simulink model "OL_HiLData"  (R2015b)
settings: Solver=FixedStepDiscrete  StartTime=0.0  StopTime=stop_time  FixedStep=step_size  RelTol=1e-3
values from neighbouring files (symbols this model uses):
  step_size = 0.1    [loadCalib.m]
  stop_time = 660    [run_test_cases.m]
undefined symbols (not defined in the file or in its folder): canChannel
libraries: canmsglib x62, canlib x29, realtime_pacer_lib x1
(part 4 of 4)

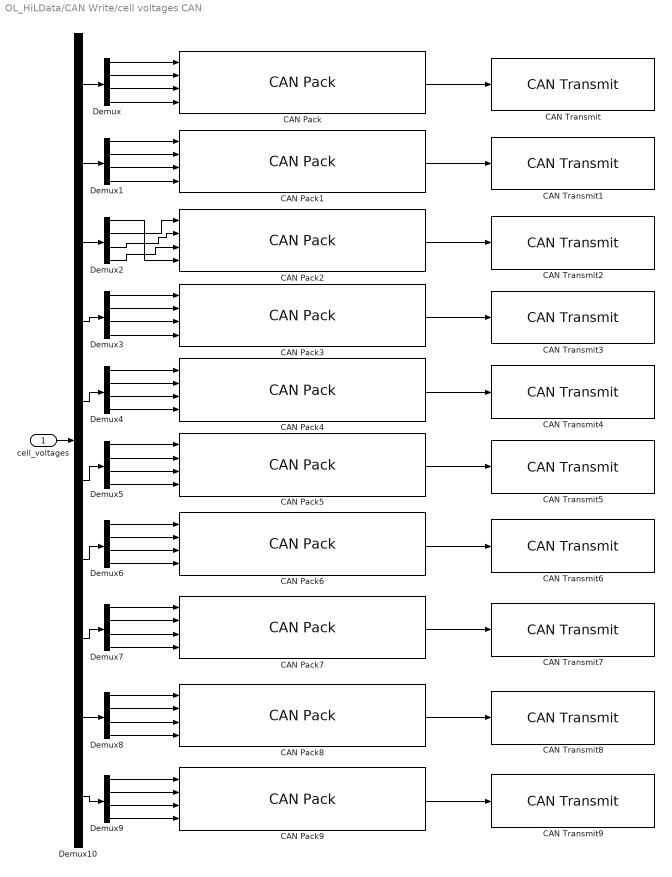
== system OL_HiLData/CAN Write/cell voltages CAN ==
  cell_voltages : Inport
  CAN Pack : canmsglib/CAN Pack  CANdbFile=D:\Projects\BMS\P006n\08_Work_in_progress\Repo_Sync_folder\OpenLoopDataSendCAN\BMSdb.dbc  MsgList=cell_voltage_1_4  MsgName=cell_voltage_1_4  MsgIDType=Standard (11-bit identifier)  MsgIdentifier=2  MsgLength=8  SignalInfo=cell1_voltage$8$16$2$2$1$0$1.000000e-04$0$0$5$#cell2_voltage$24$16$2$2$1$0$1.000000e-04$0$0$5$#cell3_voltage$40$16$2$2$1$0$1.000000e-04$0$0$5$#cell4_voltage$56$16$2$2$1$0$1.000000e-04$0$0$5$#  NSignals=4  StartBits=str2num('[int32(8);int32(24);int32(40);int32(56)]')  SignalSizes=str2num('[int32(16);int32(16);int32(16);int32(16)]')  ByteOrders=str2num('[int32(2);int32(2);int32(2);int32(2)]')  DataTypes=str2num('[int32(2);int32(2);int32(2);int32(2)]')  MultiplexTypes=str2num('[int32(1);int32(1);int32(1);int32(1)]')  MultiplexValues=str2num('[double(0);double(0);double(0);double(0)]')  Factors=str2num('[double(1.000000e-04);double(1.000000e-04);double(1.000000e-04);double(1.000000e-04)]')  Offsets=str2num('[double(0);double(0);double(0);double(0)]')  Minimums=str2num('[double(0);double(0);double(0);double(0)]')  Maximums=str2num('[double(5);double(5);double(5);double(5)]')  Remote=off
      settings: DataFormat=CANdb specified signals
  CAN Pack1 : canmsglib/CAN Pack  CANdbFile=D:\Projects\BMS\P006n\08_Work_in_progress\Repo_Sync_folder\OpenLoopDataSendCAN\BMSdb.dbc  MsgList=cell_voltage_5_8  MsgName=cell_voltage_5_8  MsgIDType=Standard (11-bit identifier)  MsgIdentifier=3  MsgLength=8  SignalInfo=cell5_votlage$8$16$2$2$1$0$1.000000e-04$0$0$5$#cell6_voltage$24$16$2$2$1$0$1.000000e-04$0$0$5$#cell7_voltage$40$16$2$2$1$0$1.000000e-04$0$0$5$#cell8_voltage$56$16$2$2$1$0$1.000000e-04$0$0$5$#  NSignals=4  StartBits=str2num('[int32(8);int32(24);int32(40);int32(56)]')  SignalSizes=str2num('[int32(16);int32(16);int32(16);int32(16)]')  ByteOrders=str2num('[int32(2);int32(2);int32(2);int32(2)]')  DataTypes=str2num('[int32(2);int32(2);int32(2);int32(2)]')  MultiplexTypes=str2num('[int32(1);int32(1);int32(1);int32(1)]')  MultiplexValues=str2num('[double(0);double(0);double(0);double(0)]')  Factors=str2num('[double(1.000000e-04);double(1.000000e-04);double(1.000000e-04);double(1.000000e-04)]')  Offsets=str2num('[double(0);double(0);double(0);double(0)]')  Minimums=str2num('[double(0);double(0);double(0);double(0)]')  Maximums=str2num('[double(5);double(5);double(5);double(5)]')  Remote=off
      settings: DataFormat=CANdb specified signals
  CAN Pack2 : canmsglib/CAN Pack  CANdbFile=D:\Projects\BMS\P006n\08_Work_in_progress\Repo_Sync_folder\OpenLoopDataSendCAN\BMSdb.dbc  MsgList=cell_voltage_9_12  MsgName=cell_voltage_9_12  MsgIDType=Standard (11-bit identifier)  MsgIdentifier=4  MsgLength=8  SignalInfo=cell10_voltage$24$16$2$2$1$0$1.000000e-04$0$0$5$#cell11_voltage$40$16$2$2$1$0$1.000000e-04$0$0$5$#cell12_voltage$56$16$2$2$1$0$1.000000e-04$0$0$5$#cell9_votlage$8$16$2$2$1$0$1.000000e-04$0$0$5$#  NSignals=4  StartBits=str2num('[int32(24);int32(40);int32(56);int32(8)]')  SignalSizes=str2num('[int32(16);int32(16);int32(16);int32(16)]')  ByteOrders=str2num('[int32(2);int32(2);int32(2);int32(2)]')  DataTypes=str2num('[int32(2);int32(2);int32(2);int32(2)]')  MultiplexTypes=str2num('[int32(1);int32(1);int32(1);int32(1)]')  MultiplexValues=str2num('[double(0);double(0);double(0);double(0)]')  Factors=str2num('[double(1.000000e-04);double(1.000000e-04);double(1.000000e-04);double(1.000000e-04)]')  Offsets=str2num('[double(0);double(0);double(0);double(0)]')  Minimums=str2num('[double(0);double(0);double(0);double(0)]')  Maximums=str2num('[double(5);double(5);double(5);double(5)]')  Remote=off
      settings: DataFormat=CANdb specified signals
  CAN Pack3 : canmsglib/CAN Pack  CANdbFile=D:\Projects\BMS\P006n\08_Work_in_progress\Repo_Sync_folder\OpenLoopDataSendCAN\BMSdb.dbc  MsgList=cell_voltage_13_16  MsgName=cell_voltage_13_16  MsgIDType=Standard (11-bit identifier)  MsgIdentifier=5  MsgLength=8  SignalInfo=cell13_votlage$8$16$2$2$1$0$1.000000e-04$0$0$5$#cell14_voltage$24$16$2$2$1$0$1.000000e-04$0$0$5$#cell15_voltage$40$16$2$2$1$0$1.000000e-04$0$0$5$#cell16_voltage$56$16$2$2$1$0$1.000000e-04$0$0$5$#  NSignals=4  StartBits=str2num('[int32(8);int32(24);int32(40);int32(56)]')  SignalSizes=str2num('[int32(16);int32(16);int32(16);int32(16)]')  ByteOrders=str2num('[int32(2);int32(2);int32(2);int32(2)]')  DataTypes=str2num('[int32(2);int32(2);int32(2);int32(2)]')  MultiplexTypes=str2num('[int32(1);int32(1);int32(1);int32(1)]')  MultiplexValues=str2num('[double(0);double(0);double(0);double(0)]')  Factors=str2num('[double(1.000000e-04);double(1.000000e-04);double(1.000000e-04);double(1.000000e-04)]')  Offsets=str2num('[double(0);double(0);double(0);double(0)]')  Minimums=str2num('[double(0);double(0);double(0);double(0)]')  Maximums=str2num('[double(5);double(5);double(5);double(5)]')  Remote=off
      settings: DataFormat=CANdb specified signals
  CAN Pack4 : canmsglib/CAN Pack  CANdbFile=D:\Projects\BMS\P006n\08_Work_in_progress\Repo_Sync_folder\OpenLoopDataSendCAN\BMSdb.dbc  MsgList=cell_voltage_17_20  MsgName=cell_voltage_17_20  MsgIDType=Standard (11-bit identifier)  MsgIdentifier=6  MsgLength=8  SignalInfo=cell17_votlage$8$16$2$2$1$0$1.000000e-04$0$0$5$#cell18_voltage$24$16$2$2$1$0$1.000000e-04$0$0$5$#cell19_voltage$40$16$2$2$1$0$1.000000e-04$0$0$5$#cell20_voltage$56$16$2$2$1$0$1.000000e-04$0$0$5$#  NSignals=4  StartBits=str2num('[int32(8);int32(24);int32(40);int32(56)]')  SignalSizes=str2num('[int32(16);int32(16);int32(16);int32(16)]')  ByteOrders=str2num('[int32(2);int32(2);int32(2);int32(2)]')  DataTypes=str2num('[int32(2);int32(2);int32(2);int32(2)]')  MultiplexTypes=str2num('[int32(1);int32(1);int32(1);int32(1)]')  MultiplexValues=str2num('[double(0);double(0);double(0);double(0)]')  Factors=str2num('[double(1.000000e-04);double(1.000000e-04);double(1.000000e-04);double(1.000000e-04)]')  Offsets=str2num('[double(0);double(0);double(0);double(0)]')  Minimums=str2num('[double(0);double(0);double(0);double(0)]')  Maximums=str2num('[double(5);double(5);double(5);double(5)]')  Remote=off
      settings: DataFormat=CANdb specified signals
  CAN Pack5 : canmsglib/CAN Pack  CANdbFile=D:\Projects\BMS\P006n\08_Work_in_progress\Repo_Sync_folder\OpenLoopDataSendCAN\BMSdb.dbc  MsgList=cell_voltage_21_24  MsgName=cell_voltage_21_24  MsgIDType=Standard (11-bit identifier)  MsgIdentifier=7  MsgLength=8  SignalInfo=cell21_votlage$8$16$2$2$1$0$1.000000e-04$0$0$5$#cell22_votlage$24$16$2$2$1$0$1.000000e-04$0$0$5$#cell23_votlage$40$16$2$2$1$0$1.000000e-04$0$0$5$#cell24_votlage$56$16$2$2$1$0$1.000000e-04$0$0$5$#  NSignals=4  StartBits=str2num('[int32(8);int32(24);int32(40);int32(56)]')  SignalSizes=str2num('[int32(16);int32(16);int32(16);int32(16)]')  ByteOrders=str2num('[int32(2);int32(2);int32(2);int32(2)]')  DataTypes=str2num('[int32(2);int32(2);int32(2);int32(2)]')  MultiplexTypes=str2num('[int32(1);int32(1);int32(1);int32(1)]')  MultiplexValues=str2num('[double(0);double(0);double(0);double(0)]')  Factors=str2num('[double(1.000000e-04);double(1.000000e-04);double(1.000000e-04);double(1.000000e-04)]')  Offsets=str2num('[double(0);double(0);double(0);double(0)]')  Minimums=str2num('[double(0);double(0);double(0);double(0)]')  Maximums=str2num('[double(5);double(5);double(5);double(5)]')  Remote=off
      settings: DataFormat=CANdb specified signals
  CAN Pack6 : canmsglib/CAN Pack  CANdbFile=D:\Projects\BMS\P006n\08_Work_in_progress\Repo_Sync_folder\OpenLoopDataSendCAN\BMSdb.dbc  MsgList=cell_voltage_25_28  MsgName=cell_voltage_25_28  MsgIDType=Standard (11-bit identifier)  MsgIdentifier=8  MsgLength=8  SignalInfo=cell25_votlage$8$16$2$2$1$0$1.000000e-04$0$0$5$#cell26_votlage$24$16$2$2$1$0$1.000000e-04$0$0$5$#cell27_votlage$40$16$2$2$1$0$1.000000e-04$0$0$5$#cell28_votlage$56$16$2$2$1$0$1.000000e-04$0$0$5$#  NSignals=4  StartBits=str2num('[int32(8);int32(24);int32(40);int32(56)]')  SignalSizes=str2num('[int32(16);int32(16);int32(16);int32(16)]')  ByteOrders=str2num('[int32(2);int32(2);int32(2);int32(2)]')  DataTypes=str2num('[int32(2);int32(2);int32(2);int32(2)]')  MultiplexTypes=str2num('[int32(1);int32(1);int32(1);int32(1)]')  MultiplexValues=str2num('[double(0);double(0);double(0);double(0)]')  Factors=str2num('[double(1.000000e-04);double(1.000000e-04);double(1.000000e-04);double(1.000000e-04)]')  Offsets=str2num('[double(0);double(0);double(0);double(0)]')  Minimums=str2num('[double(0);double(0);double(0);double(0)]')  Maximums=str2num('[double(5);double(5);double(5);double(5)]')  Remote=off
      settings: DataFormat=CANdb specified signals
  CAN Pack7 : canmsglib/CAN Pack  CANdbFile=D:\Projects\BMS\P006n\08_Work_in_progress\Repo_Sync_folder\OpenLoopDataSendCAN\BMSdb.dbc  MsgList=cell_voltage_29_32  MsgName=cell_voltage_29_32  MsgIDType=Standard (11-bit identifier)  MsgIdentifier=9  MsgLength=8  SignalInfo=cell29_votlage$8$16$2$2$1$0$1.000000e-04$0$0$5$#cell30_votlage$24$16$2$2$1$0$1.000000e-04$0$0$5$#cell31_votlage$40$16$2$2$1$0$1.000000e-04$0$0$5$#cell32_votlage$56$16$2$2$1$0$1.000000e-04$0$0$5$#  NSignals=4  StartBits=str2num('[int32(8);int32(24);int32(40);int32(56)]')  SignalSizes=str2num('[int32(16);int32(16);int32(16);int32(16)]')  ByteOrders=str2num('[int32(2);int32(2);int32(2);int32(2)]')  DataTypes=str2num('[int32(2);int32(2);int32(2);int32(2)]')  MultiplexTypes=str2num('[int32(1);int32(1);int32(1);int32(1)]')  MultiplexValues=str2num('[double(0);double(0);double(0);double(0)]')  Factors=str2num('[double(1.000000e-04);double(1.000000e-04);double(1.000000e-04);double(1.000000e-04)]')  Offsets=str2num('[double(0);double(0);double(0);double(0)]')  Minimums=str2num('[double(0);double(0);double(0);double(0)]')  Maximums=str2num('[double(5);double(5);double(5);double(5)]')  Remote=off
      settings: DataFormat=CANdb specified signals
  CAN Pack8 : canmsglib/CAN Pack  CANdbFile=D:\Projects\BMS\P006n\08_Work_in_progress\Repo_Sync_folder\OpenLoopDataSendCAN\BMSdb.dbc  MsgList=cell_voltage_33_36  MsgName=cell_voltage_33_36  MsgIDType=Standard (11-bit identifier)  MsgIdentifier=16  MsgLength=8  SignalInfo=cell33_votlage$8$16$2$2$1$0$1.000000e-04$0$0$5$#cell34_votlage$24$16$2$2$1$0$1.000000e-04$0$0$5$#cell35_votlage$40$16$2$2$1$0$1.000000e-04$0$0$5$#cell36_votlage$56$16$2$2$1$0$1.000000e-04$0$0$5$#  NSignals=4  StartBits=str2num('[int32(8);int32(24);int32(40);int32(56)]')  SignalSizes=str2num('[int32(16);int32(16);int32(16);int32(16)]')  ByteOrders=str2num('[int32(2);int32(2);int32(2);int32(2)]')  DataTypes=str2num('[int32(2);int32(2);int32(2);int32(2)]')  MultiplexTypes=str2num('[int32(1);int32(1);int32(1);int32(1)]')  MultiplexValues=str2num('[double(0);double(0);double(0);double(0)]')  Factors=str2num('[double(1.000000e-04);double(1.000000e-04);double(1.000000e-04);double(1.000000e-04)]')  Offsets=str2num('[double(0);double(0);double(0);double(0)]')  Minimums=str2num('[double(0);double(0);double(0);double(0)]')  Maximums=str2num('[double(5);double(5);double(5);double(5)]')  Remote=off
      settings: DataFormat=CANdb specified signals
  CAN Pack9 : canmsglib/CAN Pack  CANdbFile=D:\Projects\BMS\P006n\08_Work_in_progress\Repo_Sync_folder\OpenLoopDataSendCAN\BMSdb.dbc  MsgList=cell_voltage_37_40  MsgName=cell_voltage_37_40  MsgIDType=Standard (11-bit identifier)  MsgIdentifier=17  MsgLength=8  SignalInfo=cell37_votlage$8$16$2$2$1$0$1.000000e-04$0$0$5$#cell38_votlage$24$16$2$2$1$0$1.000000e-04$0$0$5$#cell39_votlage$40$16$2$2$1$0$1.000000e-04$0$0$5$#cell40_votlage$56$16$2$2$1$0$1.000000e-04$0$0$5$#  NSignals=4  StartBits=str2num('[int32(8);int32(24);int32(40);int32(56)]')  SignalSizes=str2num('[int32(16);int32(16);int32(16);int32(16)]')  ByteOrders=str2num('[int32(2);int32(2);int32(2);int32(2)]')  DataTypes=str2num('[int32(2);int32(2);int32(2);int32(2)]')  MultiplexTypes=str2num('[int32(1);int32(1);int32(1);int32(1)]')  MultiplexValues=str2num('[double(0);double(0);double(0);double(0)]')  Factors=str2num('[double(1.000000e-04);double(1.000000e-04);double(1.000000e-04);double(1.000000e-04)]')  Offsets=str2num('[double(0);double(0);double(0);double(0)]')  Minimums=str2num('[double(0);double(0);double(0);double(0)]')  Maximums=str2num('[double(5);double(5);double(5);double(5)]')  Remote=off
      settings: DataFormat=CANdb specified signals
  CAN Transmit : canlib/CAN Transmit  BlockHandle=691.0005  DeviceMenu=Kvaser Leaf Light v2 1 (Channel 1)  Device=Kvaser Leaf Light v2 1 (Channel 1)  ObjConstructor=canChannel('Kvaser', 'Leaf Light v2 1', 1)  EnablePeriodicTransmit=off  MessagePeriod=1.000
  CAN Transmit1 : canlib/CAN Transmit  BlockHandle=692.0005  DeviceMenu=Kvaser Leaf Light v2 1 (Channel 1)  Device=Kvaser Leaf Light v2 1 (Channel 1)  ObjConstructor=canChannel('Kvaser', 'Leaf Light v2 1', 1)  EnablePeriodicTransmit=off  MessagePeriod=1.000
  CAN Transmit2 : canlib/CAN Transmit  BlockHandle=693.0005  DeviceMenu=Kvaser Leaf Light v2 1 (Channel 1)  Device=Kvaser Leaf Light v2 1 (Channel 1)  ObjConstructor=canChannel('Kvaser', 'Leaf Light v2 1', 1)  EnablePeriodicTransmit=off  MessagePeriod=1.000
  CAN Transmit3 : canlib/CAN Transmit  BlockHandle=694.0005  DeviceMenu=Kvaser Leaf Light v2 1 (Channel 1)  Device=Kvaser Leaf Light v2 1 (Channel 1)  ObjConstructor=canChannel('Kvaser', 'Leaf Light v2 1', 1)  EnablePeriodicTransmit=off  MessagePeriod=1.000
  CAN Transmit4 : canlib/CAN Transmit  BlockHandle=695.0005  DeviceMenu=Kvaser Leaf Light v2 1 (Channel 1)  Device=Kvaser Leaf Light v2 1 (Channel 1)  ObjConstructor=canChannel('Kvaser', 'Leaf Light v2 1', 1)  EnablePeriodicTransmit=off  MessagePeriod=1.000
  CAN Transmit5 : canlib/CAN Transmit  BlockHandle=696.0005  DeviceMenu=Kvaser Leaf Light v2 1 (Channel 1)  Device=Kvaser Leaf Light v2 1 (Channel 1)  ObjConstructor=canChannel('Kvaser', 'Leaf Light v2 1', 1)  EnablePeriodicTransmit=off  MessagePeriod=1.000
  CAN Transmit6 : canlib/CAN Transmit  BlockHandle=697.0005  DeviceMenu=Kvaser Leaf Light v2 1 (Channel 1)  Device=Kvaser Leaf Light v2 1 (Channel 1)  ObjConstructor=canChannel('Kvaser', 'Leaf Light v2 1', 1)  EnablePeriodicTransmit=off  MessagePeriod=1.000
  CAN Transmit7 : canlib/CAN Transmit  BlockHandle=698.0005  DeviceMenu=Kvaser Leaf Light v2 1 (Channel 1)  Device=Kvaser Leaf Light v2 1 (Channel 1)  ObjConstructor=canChannel('Kvaser', 'Leaf Light v2 1', 1)  EnablePeriodicTransmit=off  MessagePeriod=1.000
  CAN Transmit8 : canlib/CAN Transmit  BlockHandle=699.0005  DeviceMenu=Kvaser Leaf Light v2 1 (Channel 1)  Device=Kvaser Leaf Light v2 1 (Channel 1)  ObjConstructor=canChannel('Kvaser', 'Leaf Light v2 1', 1)  EnablePeriodicTransmit=off  MessagePeriod=1.000
  CAN Transmit9 : canlib/CAN Transmit  BlockHandle=700.0005  DeviceMenu=Kvaser Leaf Light v2 1 (Channel 1)  Device=Kvaser Leaf Light v2 1 (Channel 1)  ObjConstructor=canChannel('Kvaser', 'Leaf Light v2 1', 1)  EnablePeriodicTransmit=off  MessagePeriod=1.000
  Demux{,1..9} (10 alike) : Demux
  Demux10 : Demux  Outputs=10
  wires:
  Demux5/4 -> CAN Pack5/4
  Demux5/1 -> CAN Pack5/1
  Demux5/2 -> CAN Pack5/2
  Demux5/3 -> CAN Pack5/3
  CAN Pack5/1 -> CAN Transmit5/1
  CAN Pack9/1 -> CAN Transmit9/1
  Demux9/4 -> CAN Pack9/4
  Demux9/1 -> CAN Pack9/1
  Demux9/2 -> CAN Pack9/2
  Demux8/1 -> CAN Pack8/1
  CAN Pack8/1 -> CAN Transmit8/1
  Demux8/3 -> CAN Pack8/3
  Demux8/2 -> CAN Pack8/2
  Demux8/4 -> CAN Pack8/4
  CAN Pack2/1 -> CAN Transmit2/1
  Demux1/4 -> CAN Pack1/4
  CAN Pack1/1 -> CAN Transmit1/1
  Demux1/1 -> CAN Pack1/1
  Demux1/2 -> CAN Pack1/2
  Demux1/3 -> CAN Pack1/3
  Demux4/1 -> CAN Pack4/1
  CAN Pack4/1 -> CAN Transmit4/1
  Demux4/3 -> CAN Pack4/3
  Demux4/2 -> CAN Pack4/2
  Demux4/4 -> CAN Pack4/4
  CAN Pack/1 -> CAN Transmit/1
  Demux/2 -> CAN Pack/2
  Demux/3 -> CAN Pack/3
  Demux/4 -> CAN Pack/4
  Demux6/2 -> CAN Pack6/2
  Demux6/4 -> CAN Pack6/4
  Demux6/3 -> CAN Pack6/3
  CAN Pack6/1 -> CAN Transmit6/1
  Demux6/1 -> CAN Pack6/1
  Demux3/2 -> CAN Pack3/2
  Demux3/1 -> CAN Pack3/1
  CAN Pack3/1 -> CAN Transmit3/1
  Demux3/4 -> CAN Pack3/4
  Demux3/3 -> CAN Pack3/3
  Demux7/2 -> CAN Pack7/2
  Demux7/4 -> CAN Pack7/4
  Demux7/3 -> CAN Pack7/3
  Demux7/1 -> CAN Pack7/1
  CAN Pack7/1 -> CAN Transmit7/1
  Demux10/1 -> Demux/1
  Demux10/2 -> Demux1/1
  Demux10/3 -> Demux2/1
  Demux10/4 -> Demux3/1
  Demux10/5 -> Demux4/1
  Demux10/6 -> Demux5/1
  Demux10/7 -> Demux6/1
  Demux10/8 -> Demux7/1
  Demux10/9 -> Demux8/1
  Demux10/10 -> Demux9/1
  cell_voltages/1 -> Demux10/1
  Demux/1 -> CAN Pack/1
  Demux9/3 -> CAN Pack9/3
  Demux2/1 -> CAN Pack2/4
  Demux2/2 -> CAN Pack2/1
  Demux2/3 -> CAN Pack2/2
  Demux2/4 -> CAN Pack2/3
